simulink model "FM_V6_Zikun"  (R2022b)
settings: Solver=VariableStepAuto  StartTime=0.0  StopTime=1240
values from neighbouring files (symbols this model uses):
  A_fc = 550    [CNV.m]
  A_st = 1.1*A_fc*1E-4*n_cell*0.0012    (= 0.047553)    [CNV.m]
  A_T_rm = 0.005    [CNV.m]
  b11 = 0.005139    [CNV.m]
  b12 = 0.00326    [CNV.m]
  b2 = 350    [CNV.m]
  c1 = 10    [CNV.m]
  c3 = 2    [CNV.m]
  cc = 30    [CNV.m]
  Cd_rm = 0.0124    [CNV.m]
  Cp_air = 1005    [CNV.m]
  Cp_cl = 4180    [CNV.m]
  Cp_st = Cp_Al*1.5    (= 1350)    [CNV.m]
  F = 96485    [CNV.m]
  gamma = 1.4    [CNV.m]
  H_conv_st = 3    [CNV.m]
  i_max = 2.2    [CNV.m]
  k_ca_out = 0.2177*10^(-5)    (= 2.177e-06)    [CNV.m]
  K_sm_out = 0.3629*10^-5    (= 3.629e-06)    [CNV.m]
  kd_cp = 0.01    [CNV.m]
  kd_rm = 0    [CNV.m]
  ki_cp = 0.1    [CNV.m]
  ki_fan = -1E-5    (= -1e-05)    [CNV.m]
  ki_rm = -5E-8    (= -5e-08)    [CNV.m]
  kp_cp = 7.5    [CNV.m]
  kp_fan = -0.5    [CNV.m]
  kp_rm = -8E-7    (= -8e-07)    [CNV.m]
  M_a = 29*10^-3    (= 0.029)    [CNV.m]
  M_H2 = 2*10^-3    (= 0.002)    [CNV.m]
  m_H2_initial = P_atm*V_an/(R_H2*T_atm)    (= 0.00044494386048)    [CNV.m]
  m_H2O_initial = 0.005    [CNV.m]
  M_m_dry = 1.1    [CNV.m]
  M_N2 = 28*10^-3    (= 0.028)    [CNV.m]
  m_N2_initial = P_atm*(1-y_O2)*V_ca/(R_N2*T_atm)    (= 0.00586138039643)    [CNV.m]
  M_O2 = 32*10^-3    (= 0.032)    [CNV.m]
  m_O2_initial = P_atm*y_O2*V_ca/(R_O2*T_atm)    (= 0.00177998712422)    [CNV.m]
  m_st = n_cell*A_fc*t_m*rho_m_dry+(V_ca+V_an)*rho_Al*2.5    (= 87.4506875)    [CNV.m]
  M_v = 18*10^-3    (= 0.018)    [CNV.m]
  n_cell = 655    [CNV.m]
  P_a = P_atm*(1-L*h/T_atm)^(g*M_a/(R*L))    [CNV.m]
  P_atm = 101.25*10^3    (= 101250)    [CNV.m]
  P_ca_ref = 2.5*P_a    [CNV.m]
  phi_a = 0.1    [CNV.m]
  phi_des = 1    [CNV.m]
  R = 8.315    [CNV.m]
  R_a = 286.9    [CNV.m]
  R_H2 = 4124.3    [CNV.m]
  R_N2 = 296.8    [CNV.m]
  R_O2 = 259.8    [CNV.m]
  R_v = 461.5    [CNV.m]
  rho_a = P_a/(R_a*T_a)    [CNV.m]
  rho_H2 = 0.0899    [CNV.m]
  rho_m_dry = 0.002    [CNV.m]
  rho_N2 = 1.165    [CNV.m]
  T_a = T_atm-h*L    [CNV.m]
  T_atm = 298.15    [CNV.m]
  T_cl = 353.15    [CNV.m]
  t_m = 0.01    [CNV.m]
  T_rm = 303.15    [CNV.m]
  T_st_ref = 353.15    [CNV.m]
  V_an = n_cell*A_fc*10^(-4)*0.0005*0.3    (= 0.00540375)    [CNV.m]
  V_ca = n_cell*A_fc*10^(-4)*0.0006*0.3    (= 0.0064845)    [CNV.m]
  V_rm = 0.005    [CNV.m]
  V_sm = 0.02    [CNV.m]
  y_O2_ca_in = 0.21    [CNV.m]
libraries: fl_lib x64, nesl_utility x40, ee_lib x18, fl_ps_legacy_lib x6, SimscapeFluids_lib x5, slpidlib x4, simulink x3, batteryecm_lib x1, autolibshared x1
(part 6 of 6)

== matlab function FM_V6_Zikun/Subsystem/FuelCellStack1/Anode Flow Model/OutletFlow/3,66a ==
  data: P_v_an input; w_an_out output; P_H2_an input; M_v input; M_H2 input
function w_an_out = fcn(P_v_an, P_H2_an,M_v,M_H2)

w_an_out = (M_v*P_v_an)/(M_H2*P_H2_an) ;

== matlab function FM_V6_Zikun/Subsystem/FuelCellStack1/Anode Flow Model/OutletFlow/outlet hydrogen mass flow rate (3.66b) ==
  data: w_an_out input; W_H2_an_out output; W_an_out input
function W_H2_an_out = fcn(w_an_out,W_an_out)

W_H2_an_out = W_an_out/(1+w_an_out);

== matlab function FM_V6_Zikun/Subsystem/FuelCellStack1/Anode Flow Model/OutletFlow/outlet vapor mass flow rate (3.66c) ==
  data: W_an_out input; W_v_an_out output; W_H2_an_out input
function W_v_an_out = fcn(W_an_out,W_H2_an_out)

W_v_an_out = W_an_out-W_H2_an_out;

== matlab function FM_V6_Zikun/Subsystem/FuelCellStack1/Anode Flow Model/PsatCalc/PsatCalc (2.31) ==
  data: T_st input; P_sat_tst output
function P_sat_tst = fcn(T_st)

%P_sat_tst = 1000*10^(-1.69*10^(-10)*T_st^4+3.85*10^(-7)*T_st^3-3.39*10^(-4)*T_st^2+0.143*T_st-20.92);
P_sat_tst = exp(20.386-5132/T_st)*133.3;

== matlab function FM_V6_Zikun/Subsystem/FuelCellStack1/Anode Flow Model/PsatCalc/PsatCalc1 (2.31) ==
  data: T_an_in input; P_sat_t_an_in output
function P_sat_t_an_in = fcn(T_an_in)

%P_sat_t_an_in = 1000*10^(-1.69*10^(-10)*T_an_in^4+3.85*10^(-7)*T_an_in^3-3.39*10^(-4)*T_an_in^2+0.143*T_an_in-20.92);
P_sat_t_an_in = exp(20.386-5132/T_an_in)*133.3;

== matlab function FM_V6_Zikun/Subsystem/FuelCellStack1/Anode Flow Model/Subsystem1/vapor pressure (3.60) ==
  data: phi_an_in input; p_v_an_in output; p_sat_t_an_in input
function p_v_an_in = fcn(phi_an_in,p_sat_t_an_in)

p_v_an_in = phi_an_in*p_sat_t_an_in;

== matlab function FM_V6_Zikun/Subsystem/Compressor/Temperature of the air leaving the compressor (2.8)/Gain calc ==
  data: gamma input; gamma_gain output
function gamma_gain = fcn(gamma)

gamma_gain = (gamma-1)/gamma;

== matlab function FM_V6_Zikun/Subsystem/Humidifier/2.36 ==
  data: P_cl input; P_a_cl output; P_v_cl input
function P_a_cl = fcn(P_cl, P_v_cl)

P_a_cl = P_cl - P_v_cl;

== matlab function FM_V6_Zikun/Subsystem/Compressor/Temperature of the air leaving the compressor (2.8)/Temperature add ==
  data: T_atm input; T_add_cp output; eta_cp input; P_sm input; P_atm input; gamma_gain input
function T_add_cp = fcn(T_atm,eta_cp,P_sm,P_atm,gamma_gain)

T_add_cp = (T_atm/eta_cp) *( ( (P_sm/P_atm) ^ gamma_gain ) -1);

== matlab function FM_V6_Zikun/Subsystem/FuelCellStack1/Anode Flow Model/ThermodynamicCalc/3.56 ==
  data: m_H2_an input; P_H2_an output; T_st input; V_an input; R_H2 input
function P_H2_an = fcn(m_H2_an,T_st,V_an,R_H2)

P_H2_an = m_H2_an*R_H2*T_st/V_an;

== matlab function FM_V6_Zikun/Subsystem/FuelCellStack1/Anode Flow Model/ThermodynamicCalc/3.56//3.57 N2 ==
  data: m_N2_an input; P_N2_an output; T_st input; V_an input; R_N2 input
function P_N2_an = fcn(m_N2_an,T_st,V_an,R_N2)

P_N2_an = m_N2_an*R_N2*T_st/V_an;

== matlab function FM_V6_Zikun/Subsystem/FuelCellStack1/Anode Flow Model/ThermodynamicCalc/3.56//3.57 O2 ==
  data: m_O2_an input; P_O2_an output; T_st input; V_an input; R_O2 input
function P_O2_an = fcn(m_O2_an,T_st,V_an,R_O2)

P_O2_an = m_O2_an*R_O2*T_st/V_an;

== matlab function FM_V6_Zikun/Subsystem/FuelCellStack1/Anode Flow Model/ThermodynamicCalc/3.57 ==
  data: m_v_an input; P_v_an output; T_st input; V_an input; R_v input
function P_v_an = fcn(m_v_an,T_st,V_an,R_v)

P_v_an = m_v_an*R_v*T_st/V_an;

== matlab function FM_V6_Zikun/Subsystem/FuelCellStack1/CathodMassFlow/CathodMassBalance/3.25 ==
  data: W_O2_ca_in input; dm_O2_ca_in output; W_O2_ca_out input; W_O2_reac input
function dm_O2_ca_in = fcn(W_O2_ca_in,W_O2_ca_out,W_O2_reac)

dm_O2_ca_in = W_O2_ca_in-W_O2_ca_out-W_O2_reac;

== matlab function FM_V6_Zikun/Subsystem/FuelCellStack1/CathodMassFlow/CathodMassBalance/3.26 ==
  data: W_N2_ca_in input; dm_N2_ca output; W_N2_ca_out input
function dm_N2_ca= fcn(W_N2_ca_in,W_N2_ca_out)

dm_N2_ca = W_N2_ca_in-W_N2_ca_out;

== matlab function FM_V6_Zikun/Subsystem/FuelCellStack1/CathodMassFlow/CathodMassBalance/3.27 ==
  data: W_v_ca_in input; dm_w_ca output; W_v_ca_out input; W_v_ca_gen input; W_v_ca_mem input; W_l_ca_out input
function dm_w_ca = fcn(W_v_ca_in,W_v_ca_out,W_v_ca_gen,W_v_ca_mem,W_l_ca_out)

dm_w_ca = W_v_ca_in-W_v_ca_out+W_v_ca_gen+W_v_ca_mem-W_l_ca_out;

== matlab function FM_V6_Zikun/Subsystem/Supply Manifold/Manifold Filling/MATLAB Function ==
  data: W_cp input; d_m_sm_dt output; W_sm_out input
function d_m_sm_dt = fcn(W_cp, W_sm_out)

d_m_sm_dt = W_cp - W_sm_out;

== matlab function FM_V6_Zikun/Subsystem/FuelCellStack1/CathodMassFlow/CathodMassBalance/3.28 ==
  data: P_sat input; m_v_max_ca output; T_st input; V_ca input
function m_v_max_ca = fcn(P_sat,T_st,V_ca)

R_v = 461.5;
m_v_max_ca = P_sat*V_ca/(R_v*T_st);

== matlab function FM_V6_Zikun/Subsystem/FuelCellStack1/CathodMassFlow/CathodMassBalance/3.29&3.30 ==
  data: m_w_ca input; m_v_max_ca input; m_v_ca output; m_l_ca output
function [m_v_ca, m_l_ca]  = fcn(m_w_ca,m_v_max_ca)

if m_w_ca <= m_v_max_ca
    m_v_ca = m_w_ca;
else
    m_v_ca = m_v_max_ca;
end

if m_w_ca <= m_v_max_ca
    m_l_ca = 0;
else
    m_l_ca = m_w_ca-m_v_max_ca;
end

== matlab function FM_V6_Zikun/Subsystem/FuelCellStack1/CathodMassFlow/ElectroChemistry/MATLAB Function ==
  data: I_st input; W_O2_reac output; n_cell input; M_O2 input; F input
function W_O2_reac = fcn(I_st,n_cell,M_O2,F)

W_O2_reac = M_O2*n_cell*I_st/(4*F);

== matlab function FM_V6_Zikun/Subsystem/FuelCellStack1/CathodMassFlow/ElectroChemistry/MATLAB Function1 ==
  data: I_st input; W_v_gen output; n_cell input; M_v input; F input
function W_v_gen = fcn(I_st,n_cell,M_v,F)

W_v_gen = M_v*n_cell*I_st/(4*F);

== matlab function FM_V6_Zikun/Subsystem/FuelCellStack1/CathodMassFlow/InletFlowPropertiesCalc/3.40 ==
  data: w_ca_in output; M_a_ca_in input; P_v_ca_in input; P_a_ca_in input; M_v input
function w_ca_in = fcn(M_a_ca_in,P_v_ca_in,P_a_ca_in,M_v)

w_ca_in = M_v*P_v_ca_in/(M_a_ca_in*P_a_ca_in);

== matlab function FM_V6_Zikun/Subsystem/FuelCellStack1/CathodMassFlow/InletFlowPropertiesCalc/3.41 ==
  data: y_O2_ca_in input; M_a_ca_in output; M_O2 input; M_N2 input
function M_a_ca_in = fcn(y_O2_ca_in,M_O2,M_N2)

M_a_ca_in = y_O2_ca_in*M_O2+(1-y_O2_ca_in)*M_N2;

== matlab function FM_V6_Zikun/Subsystem/FuelCellStack1/CathodMassFlow/InletFlowPropertiesCalc/3.42 ==
  data: W_ca_in input; W_a_ca_in output; w_ca_in input
function W_a_ca_in = fcn(W_ca_in,w_ca_in)

W_a_ca_in = (1/(1+w_ca_in))*W_ca_in;

== matlab function FM_V6_Zikun/Subsystem/FuelCellStack1/CathodMassFlow/InletFlowPropertiesCalc/3.46 ==
  data: y_O2_ca_in input; x_O2_ca_in output; M_O2 input; M_N2 input
function x_O2_ca_in = fcn(y_O2_ca_in,M_O2,M_N2)

x_O2_ca_in = y_O2_ca_in*M_O2/(y_O2_ca_in*M_O2+(1-y_O2_ca_in)*M_N2);

== matlab function FM_V6_Zikun/Subsystem/FuelCellStack1/CathodMassFlow/Diffusion/O2 and N2 Crossflow ==
  data: n_cell input; W_O2_ca_cf output; A_fc input; t_m input; P_ca input; W_O2_ca_in input; W_N2_ca_in input; T_st input; lambda_m input; W_O2_ca_in2 output; W_N2_ca_cf output; W_N2_ca_in2 output; R input
function [W_O2_ca_cf, W_O2_ca_in2, W_N2_ca_cf, W_N2_ca_in2]= fcn(n_cell, A_fc, t_m, P_ca, W_O2_ca_in, W_N2_ca_in, T_st, lambda_m, R)

%% Oxygen Crossflow
D_O2 = 0.0031*exp(-2768/T_st); % Diffusivity, cm^2/s (4.17)
S_O2 = 7.43E-12*exp(666/T_st); % Solubility, mol/(cm^3*Pa)

Pm_O2 = D_O2*S_O2; % Permeability, mol*cm/(s*cm^2*Pa) (4.16)

K_GDL_O2 = 1;
P_O2 = P_ca*0.21*K_GDL_O2;

m_M_O2 = 31.999E-3; % Molar mass, kg/mol
W_O2_ca_cf = Pm_O2*n_cell*A_fc*P_O2/t_m*m_M_O2; % Cross flow, kg/s

W_O2_ca_in2 = W_O2_ca_in - W_O2_ca_cf; % Remaining oxygen flow

%% Nitrogen Crossflow
Vm_w = 0.018; %molar volume of water, L/mol
Vm_mem = 0.55; %molar volume of membrane
f_v = lambda_m*Vm_w/(Vm_mem+lambda_m*Vm_w);
T_ref = 303;
E_N2 = 24;

K_GDL_N2 = 1;
P_N2 = P_ca*0.78*K_GDL_N2;

alpha_N2 = 0.002; %Scale factor
Pm_N2 = alpha_N2*(0.0295+1.21*f_v-1.93*f_v^2)*10^-11*exp(E_N2/R*(1/T_ref-1/T_st)); % Permeability, kmol*cm/(s*cm^2*bar)

m_M_N2 = 28.013E-3; % Molar mass, kg/mol
W_N2_ca_cf = 1000*Pm_N2*n_cell*A_fc*(P_N2*0.78/10^5)/t_m*m_M_N2; % Cross flow, kg/s
W_N2_ca_in2 = W_N2_ca_in - W_N2_ca_cf; % Remaining nitrogen flow

== matlab function FM_V6_Zikun/Subsystem/Supply Manifold/Nozzle/MATLAB Function ==
  data: P_sm input; W_sm_out output; P_ca input; k_sm_out input
function W_sm_out = fcn(P_sm, P_ca,k_sm_out)

   % k_sm_out = 0.3629*10^-5; %kg/sPa
    W_sm_out = k_sm_out*(P_sm - P_ca);

== matlab function FM_V6_Zikun/Subsystem/AirExhaustManifold/MATLAB Function2 ==
  data: k_ca_out input; W_ca_out output; P_ca input; P_rm input
function W_ca_out = fcn(k_ca_out,P_ca,P_rm)

W_ca_out = k_ca_out*(P_ca-P_rm);

== matlab function FM_V6_Zikun/Subsystem/FuelCellStack1/CathodMassFlow/OutletFlowPropertiesCalc/3.48a ==
  data: y_O2_ca input; M_a_ca output; M_O2 input; M_N2 input
function M_a_ca = fcn(y_O2_ca,M_O2,M_N2)

M_a_ca = y_O2_ca*M_O2+(1-y_O2_ca)*M_N2;

== matlab function FM_V6_Zikun/Subsystem/FuelCellStack1/CathodMassFlow/OutletFlowPropertiesCalc/3.48b ==
  data: w_ca_out output; M_a_ca input; P_v_ca input; P_a_ca input; M_v input
function w_ca_out = fcn(M_a_ca,P_v_ca,P_a_ca,M_v)

w_ca_out = M_v*P_v_ca/(M_a_ca*P_a_ca);

== matlab function FM_V6_Zikun/Subsystem/FuelCellStack1/CathodMassFlow/OutletFlowPropertiesCalc/3.48c ==
  data: W_ca_out input; W_a_ca_out output; w_ca_out input
function W_a_ca_out = fcn(W_ca_out,w_ca_out)

W_a_ca_out = (1/(1+w_ca_out))*W_ca_out;

== matlab function FM_V6_Zikun/Subsystem/FuelCellStack1/CathodMassFlow/OutletFlowPropertiesCalc/3.48e ==
  data: y_O2_ca input; x_O2_ca output; M_O2 input; M_N2 input
function x_O2_ca = fcn(y_O2_ca,M_O2,M_N2)

x_O2_ca = y_O2_ca*M_O2/(y_O2_ca*M_O2+(1-y_O2_ca)*M_N2);

== matlab function FM_V6_Zikun/Subsystem/FuelCellStack1/CathodMassFlow/PsatCalc ==
  data: T_ca_in input; P_sat_ca_in output
function P_sat_ca_in = fcn(T_ca_in)

%P_sat_ca_in = 1000*10^(-1.69*10^(-10)*T_ca_in^4+3.85*10^(-7)*T_ca_in^3-3.39*10^(-4)*T_ca_in^2+0.143*T_ca_in-20.92);
P_sat_ca_in = exp(20.386-5132/T_ca_in)*133.3;

== matlab function FM_V6_Zikun/Subsystem/FuelCellStack1/CathodMassFlow/ThermodynamicCalc/3.31 ==
  data: m_O2_ca input; P_O2_Ca output; R_O2 input; T_st input; V_ca input
function P_O2_Ca = fcn(m_O2_ca,R_O2,T_st,V_ca)

P_O2_Ca = m_O2_ca*R_O2*T_st/V_ca;

== matlab function FM_V6_Zikun/Subsystem/FuelCellStack1/CathodMassFlow/ThermodynamicCalc/3.32 ==
  data: m_N2_ca input; P_N2_Ca output; R_N2 input; T_st input; V_ca input
function P_N2_Ca = fcn(m_N2_ca,R_N2,T_st,V_ca)

P_N2_Ca = m_N2_ca*R_N2*T_st/V_ca;

== matlab function FM_V6_Zikun/Subsystem/FuelCellStack1/CathodMassFlow/ThermodynamicCalc/3.33 ==
  data: m_v_ca input; P_v_Ca output; R_v input; T_st input; V_ca input
function P_v_Ca = fcn(m_v_ca,R_v,T_st,V_ca)

P_v_Ca = m_v_ca*R_v*T_st/V_ca;

== matlab function FM_V6_Zikun/Subsystem/Supply Manifold/Manifold Filling/MATLAB Function1 ==
  data: W_cp input; d_p_sm_dt output; T_cp_out input; W_sm_out input; T_sm input; gamma input; R_a input; V_sm input
function d_p_sm_dt = fcn(W_cp, T_cp_out, W_sm_out, T_sm,gamma,R_a,V_sm)
    %gamma = 1.4;
    %Ra = 286.9; % J/KgK
    %V_sm = 0.02;
    d_p_sm_dt = ((gamma * R_a) / V_sm) * (W_cp * T_cp_out - W_sm_out * T_sm);

== matlab function FM_V6_Zikun/Subsystem/FuelCellStack1/MembraneHydration/3.67-3.70 ==
  data: W_v_mem output; n_d input; i input; D_w input; c_v_ca input; c_v_an input; n_cell input; A_fc input; M_v input; t_m input; F input
function W_v_mem = fcn(n_d,i,D_w,c_v_ca,c_v_an,n_cell,A_fc,M_v,t_m,F)

W_v_mem = n_cell*A_fc*M_v*(n_d*i/F-D_w*(c_v_ca-c_v_an)/t_m);

== matlab function FM_V6_Zikun/Subsystem/FuelCellStack1/MembraneHydration/3.72-3.73 ==
  data: phi_ca input; lambda_m output; phi_an input; lambda_ca output; lambda_an output
function [lambda_m,lambda_ca,lambda_an] = fcn(phi_ca,phi_an)

phi_m = (phi_ca+phi_an)/2;

if phi_m <= 1
    lambda_m = 0.043+17.81*phi_m-39.85*phi_m^2+36*phi_m^3;
elseif (1 < phi_m) <=3
    lambda_m = 14+1.4*(phi_m-1);
else
    lambda_m = NaN;
end
%%
if phi_ca <= 1
    lambda_ca = 0.043+17.81*phi_ca-39.85*phi_ca^2+36*phi_ca^3;
elseif (1 < phi_ca) <=3
    lambda_ca = 14+1.4*(phi_ca-1);
else
    lambda_ca = NaN;
end
%%
if phi_an <= 1
    lambda_an = 0.043+17.81*phi_an-39.85*phi_an^2+36*phi_an^3;
elseif (1 < phi_an) <=3
    lambda_an = 14+1.4*(phi_an-1);
else
    lambda_an = NaN;
end

== matlab function FM_V6_Zikun/Subsystem/FuelCellStack1/MembraneHydration/3.74 ==
  data: lambda_m input; n_d output
function n_d = fcn(lambda_m)

n_d = 0.0029*lambda_m^2+0.05*lambda_m-3.4*10^(-19);

== matlab function FM_V6_Zikun/Subsystem/FuelCellStack1/MembraneHydration/3.75-3.76 ==
  data: lambda_m input; D_w output; T_st input
function D_w = fcn(lambda_m,T_st)

%%
if lambda_m < 2
    D_lambda = 10^(-6);
elseif (2 <= lambda_m) <= 3
    D_lambda = 10^(-6)*(1+2*(lambda_m-2));
elseif (3 < lambda_m) < 4.5
    D_lambda = 10^(-6)*(3-1.67*(lambda_m-3));
else
    D_lambda = 1.25*10^(-6);
end

%%
D_w = D_lambda*exp(2416*(1/303-1/T_st));

== matlab function FM_V6_Zikun/Subsystem/FuelCellStack1/PsatCalc ==
  data: T_st input; P_sat output
function P_sat = fcn(T_st)

%P_sat = 1000*10^(-1.69*10^(-10)*T_st^4+3.85*10^(-7)*T_st^3-3.39*10^(-4)*T_st^2+0.143*T_st-20.92);
P_sat = exp(20.386-5132/T_st)*133.3;

== matlab function FM_V6_Zikun/Subsystem/FuelCellStack1/StackVoltage/ActivationLoss/ActivitionLoss ==
  data: V0 input; V_act output; Va input; c1 input; I_den input
function V_act= fcn(V0, Va, c1, I_den)

V_act = V0+Va*(1-exp(-c1*I_den));

== matlab function FM_V6_Zikun/Subsystem/FuelCellStack1/StackVoltage/ActivationLoss/MATLAB Function ==
  data: T_st input; V0 output; P_ca input; P_sat input
function V0= fcn(T_st,P_ca,P_sat)

V0 = 0.279-8.5*10^(-4)*(T_st-298.15)+4.308*10^(-5)*T_st*(log((P_ca-P_sat)/1.01325)+0.5*log(0.1173*(P_ca-P_sat)/1.01325));

== matlab function FM_V6_Zikun/Subsystem/FuelCellStack1/StackVoltage/ActivationLoss/MATLAB Function1 ==
  data: Va output; T_st input; P_O2 input; P_sat input
function Va = fcn(T_st,P_O2,P_sat)

Va = (-1.618*10^(-5)*T_st+1.618*10^(-2))*(P_O2/0.1173+P_sat)^2+(1.8*10^(-4)*T_st-0.166)*(P_O2/0.1173+P_sat)+(-5.8*10^(-4)*T_st+0.5736);

== matlab function FM_V6_Zikun/Subsystem/FuelCellStack1/StackVoltage/ActivationLoss/MATLAB Function2 ==
  data: V0 input; R_act output; Va input; c1 input; I_den input
function R_act = fcn(V0,Va,c1,I_den)

R_act = (V0+Va*(1-exp(-c1*I_den)))/I_den;

== matlab function FM_V6_Zikun/Subsystem/FuelCellStack1/StackVoltage/ConcentrationLoss/MATLAB Function ==
  data: I_den input; V_conc output; c2 input; i_max input; c3 input
function V_conc = fcn(I_den,c2,i_max,c3)

V_conc = I_den*(c2*I_den/i_max)^c3;

== matlab function FM_V6_Zikun/Subsystem/FuelCellStack1/StackVoltage/ConcentrationLoss/MATLAB Function1 ==
  data: T_st input; c2 output; P_O2 input; P_sat input
function c2 = fcn(T_st,P_O2,P_sat)

if (P_O2/0.1173+P_sat) < 2
    c2 = (7.16*(10^-4)*T_st-0.622)*(P_O2/0.1173+P_sat)+(-1.45*10^(-3)*T_st+1.68);
else
    c2 = (8.66*(10^-5)*T_st-0.068)*(P_O2/0.1173+P_sat)+(-1.6*10^(-4)*T_st+0.54);
end

== matlab function FM_V6_Zikun/Subsystem/FuelCellStack1/StackVoltage/ConcentrationLoss/MATLAB Function2 ==
  data: c2 input; R_conc output; I_den input; i_max input; c3 input
function R_conc = fcn(c2,I_den,i_max,c3)

R_conc = (c2*I_den/i_max)^c3;

== matlab function FM_V6_Zikun/Subsystem/FuelCellStack1/StackVoltage/NernstVoltage ==
  data: T_st input; E_T_P output; P_H2 input; P_O2 input
function E_T_P = fcn(T_st, P_H2, P_O2)

E_T_P = 1.229-8.5*10^(-4)*(T_st-298.15)+4.308*10^(-5)*T_st*(log(P_H2/1.01325)+0.5*log(P_O2/1.01325));

== matlab function FM_V6_Zikun/Subsystem/Humidifier/2.37 ==
  data: P_v_cl input; weber_cl output; P_a_cl input; M_v input; M_a input
function weber_cl= fcn(P_v_cl, P_a_cl, M_v, M_a)

weber_cl = (M_v/M_a)*(P_v_cl/P_a_cl);

== matlab function FM_V6_Zikun/Subsystem/FuelCellStack1/StackVoltage/OhmicLoss/MATLAB Function ==
  data: I_den input; V_ohm output; T_st input; lambda_m input; t_m input; b11 input; b12 input; b2 input
function V_ohm = fcn(I_den,T_st,lambda_m,t_m,b11,b12,b2)

V_ohm = I_den*(t_m/((b11*lambda_m-b12)*exp(b2*(1/303-1/T_st))));

== matlab function FM_V6_Zikun/Subsystem/FuelCellStack1/Thermo/MATLAB Function ==
  data: I_st input; P_loss_reac output; V_cell input; n_cell input
function P_loss_reac = fcn(I_st,V_cell,n_cell)

P_loss_reac = n_cell*I_st*(1.482-V_cell);

== matlab function FM_V6_Zikun/Subsystem/FuelCellStack1/Anode Recirculation and Purge System1/MATLAB Function ==
  data: P_an input; T_an input; V_N2 output; m_N2 input; m_O2 input; V_O2 output; R_N2 input; R_O2 input
function [V_N2, V_O2] = fcn(P_an, T_an, m_N2, m_O2, R_N2, R_O2)

V_N2 = m_N2*R_N2*T_an/P_an;

V_O2 = m_O2*R_O2*T_an/P_an;

== matlab function FM_V6_Zikun/Subsystem/FuelCellStack1/Anode Recirculation and Purge System1/MATLAB Function1 ==
  data: V_recirc input; H2_ratio output; V_cont input
function H2_ratio = fcn(V_recirc, V_cont)

H2_ratio = (V_recirc-V_cont)/V_recirc;

== matlab function FM_V6_Zikun/Subsystem/Humidifier/2.35 ==
  data: Phi_cl input; P_v_cl output; P_sat_T_cl input
function P_v_cl = fcn(Phi_cl, P_sat_T_cl)

P_v_cl = Phi_cl * P_sat_T_cl;

== matlab function FM_V6_Zikun/Subsystem/Humidifier/2.38 ==
  data: W_cl input; W_a_cl output; weber_cl input
function W_a_cl = fcn(W_cl, weber_cl)

W_a_cl = (1/(1+weber_cl))*W_cl;
